simulink model "comprehensive_model_with_rocks_trial"  (R2019a)
settings: Solver=FixedStepAuto  StartTime=0.0  StopTime=15  FixedStep=0.001  RelTol=1e-3
PreLoadFcn:
  | load('tumbleweed_constants.mat')
values from neighbouring files (symbols this model uses):
  Ar = 0.785398163397    [tumbleweed_constants.mat]
  CD = 0.8    [tumbleweed_constants.mat]
  d = 0.65    [tumbleweed_constants.mat]
  g = 9.81    [tumbleweed_constants.mat]
  Ixx = 1.29    [tumbleweed_constants.mat]
  Iyy = 1.29    [tumbleweed_constants.mat]
  Izz = 1.29    [tumbleweed_constants.mat]
  m = 1    [tumbleweed_constants.mat]
  maxr = 0.45    [tumbleweed_constants.mat]
  mf = 14    [tumbleweed_constants.mat]
  minr = 0.2    [tumbleweed_constants.mat]
  mu0 = 0.02    [tumbleweed_constants.mat]
  muk = 0.5    [tumbleweed_constants.mat]
  must = 0.8    [tumbleweed_constants.mat]
  R = cylR*ones(size(Theta,1),size(Theta,2))    [d3_animate.m]    (also in tumbleweed_constants.mat = 0.5)
  rest_coeff = 0.6    [tumbleweed_constants.mat]
  rho = 1.2    [tumbleweed_constants.mat]
  ts = 0.5    [tumbleweed_constants.mat]
  v_thres = 0.0001    [tumbleweed_constants.mat]
  vmax = 0.2    [tumbleweed_constants.mat]
  YY = 50    [tumbleweed_constants.mat]
libraries: simulink x2
(part 1 of 9)
settings Model: Creator=racha  LastModifiedBy=racha

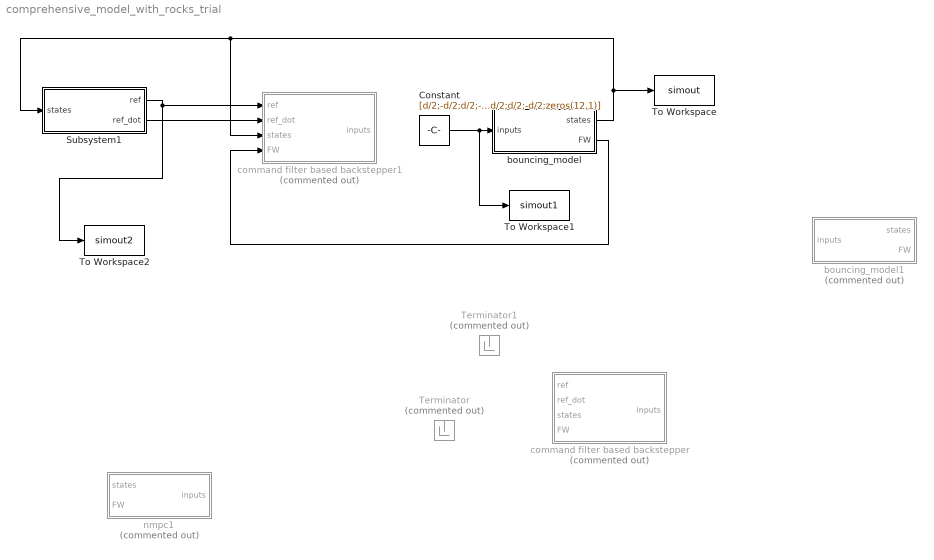
== system comprehensive_model_with_rocks_trial ==
  Constant : Constant  Value=[d/2;-d/2;d/2;-d/2;d/2;-d/2;zeros(12,1)]
  Subsystem1 : Subsystem
  Terminator : Terminator  Commented=on
  Terminator1 : Terminator  Commented=on
  To Workspace : ToWorkspace  VariableName=simout  SaveFormat=Timeseries  SampleTime=-1
  To Workspace1 : ToWorkspace  VariableName=simout1  SaveFormat=Timeseries  SampleTime=-1
  To Workspace2 : ToWorkspace  VariableName=simout2  SaveFormat=Timeseries  SampleTime=-1
  bouncing_model : Subsystem
  bouncing_model1 : Subsystem  Commented=on
  command filter based backstepper : Subsystem  Commented=on
  command filter based backstepper1 : Subsystem  Commented=on
  nmpc1 : Subsystem  Commented=on
  wires:
  bouncing_model/2(FW) -> command filter based backstepper1/4(FW)
  Subsystem1/1(ref) -> command filter based backstepper1/1(ref), To Workspace2/1
  Subsystem1/2("ref_dot ") -> command filter based backstepper1/2("ref_dot ")
  bouncing_model/1(states) -> command filter based backstepper1/3(states), Subsystem1/1(states), To Workspace/1
  Constant/1 -> To Workspace1/1, bouncing_model/1(inputs)

== system comprehensive_model_with_rocks_trial/Subsystem1 ==
  states : Inport
  Clock : Clock
  Constant : Constant  Commented=on  Value=[-0.5;-0.5;0.5]
  Data Store Memory : DataStoreMemory  DataStoreName=y_new  ReadBeforeWriteMsg=warning  WriteAfterWriteMsg=warning  WriteAfterReadMsg=warning  InitialValue=[0;0]  ShowAdditionalParam=off
  Data Store Memory1 : DataStoreMemory  DataStoreName=err  ReadBeforeWriteMsg=warning  WriteAfterWriteMsg=warning  WriteAfterReadMsg=warning  InitialValue=[0;0]  ShowAdditionalParam=off
  Data Store Memory2 : DataStoreMemory  DataStoreName=cum_err  ReadBeforeWriteMsg=warning  WriteAfterWriteMsg=warning  WriteAfterReadMsg=warning  ShowAdditionalParam=off
  Data Store Read : DataStoreRead  DataStoreName=hit
  Data Store Read1 : DataStoreRead  DataStoreName=y_new
  Data Store Read2 : DataStoreRead  DataStoreName=err
  Data Store Read3 : DataStoreRead  DataStoreName=cum_err
  Data Store Write : DataStoreWrite  DataStoreName=hit
  Data Store Write1 : DataStoreWrite  DataStoreName=y_new
  Data Store Write2 : DataStoreWrite  DataStoreName=err
  Data Store Write3 : DataStoreWrite  DataStoreName=cum_err
  MATLAB Function : MATLAB Function  TreatAsAtomicUnit=on
  Stop Simulation : Stop
  Uniform Random Number : UniformRandomNumber  Minimum=0  Seed=43  SampleTime=0.01
  t : DataStoreMemory  DataStoreName=hit  ReadBeforeWriteMsg=warning  WriteAfterWriteMsg=warning  WriteAfterReadMsg=warning  ShowAdditionalParam=off
  y_points : ToWorkspace  VariableName=simout5  SaveFormat=Timeseries  SampleTime=-1
  yref_points : ToWorkspace  VariableName=simout10  SaveFormat=Timeseries  SampleTime=-1
  ref : Outport
  "ref_dot " : Outport  Port=2
  wires:
  MATLAB Function/1(y) -> ref/1
  Clock/1 -> MATLAB Function/1(t)
  MATLAB Function/2(ydot) -> "ref_dot "/1
  states/1 -> MATLAB Function/2(states)
  Data Store Read/1 -> MATLAB Function/3("hit ")
  MATLAB Function/3(hit) -> Data Store Write/1
  Data Store Read1/1 -> MATLAB Function/4("y_new ")
  MATLAB Function/4(y_new) -> Data Store Write1/1, yref_points/1
  Data Store Read2/1 -> MATLAB Function/5("err ")
  Data Store Read3/1 -> MATLAB Function/6("cum_err ")
  MATLAB Function/5(err) -> y_points/1, Data Store Write2/1
  MATLAB Function/6(cum_err) -> Data Store Write3/1
  Uniform Random Number/1 -> MATLAB Function/7(rand_num)
  MATLAB Function/7(stop_flag) -> Stop Simulation/1

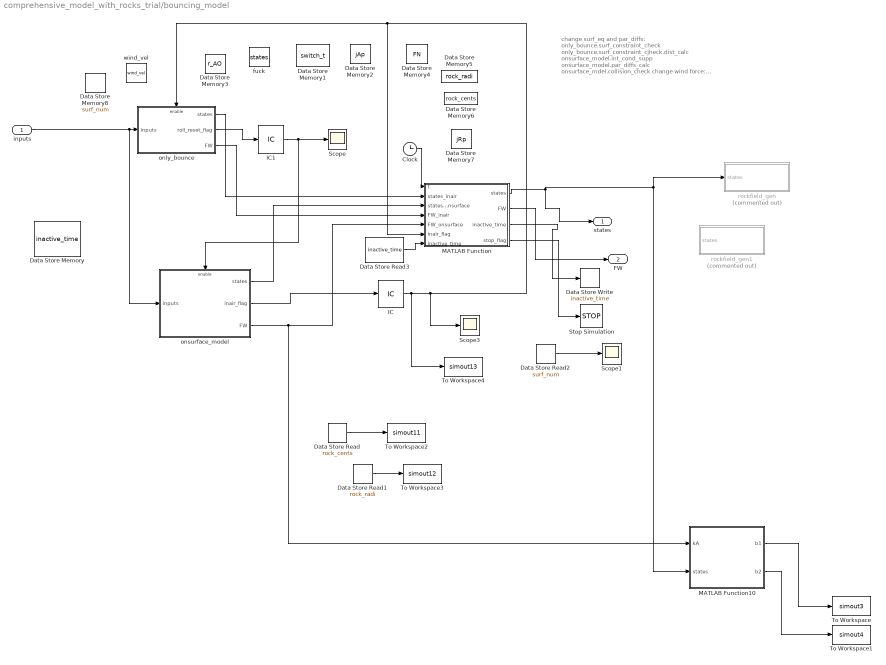
== system comprehensive_model_with_rocks_trial/bouncing_model ==
  note: change surf_eq and par_diffs:
      | only_bounce.surf_constraint_check
      | only_bounce.surf_constraint_cjheck.dist_calc
      | onsurface_model.int_cond_supp
      | onsurface_model.par_diffs_calc
      | onsurface_mdel.collision_check
      |
      | change wind force:
      | only_bounce.wind_force_calc
      | onsurface_model.wind_force_calc
      |
      | FN = 0 only when u start from surface
  inputs : Inport
  Clock : Clock
  Data Store Memory : DataStoreMemory  DataStoreName=inactive_time  ReadBeforeWriteMsg=warning  WriteAfterWriteMsg=warning  WriteAfterReadMsg=warning  ShowAdditionalParam=off
  Data Store Memory1 : DataStoreMemory  DataStoreName=switch_t  ReadBeforeWriteMsg=warning  WriteAfterWriteMsg=warning  WriteAfterReadMsg=warning  ShowAdditionalParam=off
  Data Store Memory2 : DataStoreMemory  DataStoreName=jAp  ReadBeforeWriteMsg=warning  WriteAfterWriteMsg=warning  WriteAfterReadMsg=warning  InitialValue=[0;1;0]  ShowAdditionalParam=off
  Data Store Memory3 : DataStoreMemory  DataStoreName=r_AO  ReadBeforeWriteMsg=warning  WriteAfterWriteMsg=warning  WriteAfterReadMsg=warning  InitialValue=[0;0;0]  ShowAdditionalParam=off
  Data Store Memory4 : DataStoreMemory  DataStoreName=FN  ReadBeforeWriteMsg=warning  WriteAfterWriteMsg=warning  WriteAfterReadMsg=warning  InitialValue=100  ShowAdditionalParam=off
  Data Store Memory5 : DataStoreMemory  DataStoreName=rock_radi  ReadBeforeWriteMsg=warning  WriteAfterWriteMsg=warning  WriteAfterReadMsg=warning  InitialValue=[0.2;0.5]  ShowAdditionalParam=off
  Data Store Memory6 : DataStoreMemory  DataStoreName=rock_cents  ReadBeforeWriteMsg=warning  WriteAfterWriteMsg=warning  WriteAfterReadMsg=warning  InitialValue=[5,7;0,0;-0.1,-0.1]  ShowAdditionalParam=off
  Data Store Memory7 : DataStoreMemory  DataStoreName=jRp  ReadBeforeWriteMsg=warning  WriteAfterWriteMsg=warning  WriteAfterReadMsg=warning  InitialValue=[0;1;0]  ShowAdditionalParam=off
  Data Store Memory8 : DataStoreMemory  DataStoreName=surf_num  ReadBeforeWriteMsg=warning  WriteAfterWriteMsg=warning  WriteAfterReadMsg=warning  ShowAdditionalParam=off
  Data Store Read : DataStoreRead  DataStoreName=rock_cents
  Data Store Read1 : DataStoreRead  DataStoreName=rock_radi
  Data Store Read2 : DataStoreRead  DataStoreName=surf_num
  Data Store Read3 : DataStoreRead  DataStoreName=inactive_time
  Data Store Write : DataStoreWrite  DataStoreName=inactive_time
  IC : InitialCondition
  IC1 : InitialCondition  Value=0
  MATLAB Function : MATLAB Function  TreatAsAtomicUnit=on
  MATLAB Function10 : MATLAB Function  TreatAsAtomicUnit=on
  Scope : Scope
  Scope1 : Scope
  Scope3 : Scope
  Stop Simulation : Stop
  To Workspace : ToWorkspace  VariableName=simout3  SaveFormat=Timeseries  SampleTime=-1
  To Workspace1 : ToWorkspace  VariableName=simout4  SaveFormat=Timeseries  SampleTime=-1
  To Workspace2 : ToWorkspace  VariableName=simout11  SaveFormat=Timeseries  SampleTime=-1
  To Workspace3 : ToWorkspace  VariableName=simout12  SaveFormat=Timeseries  SampleTime=-1
  To Workspace4 : ToWorkspace  VariableName=simout13  SaveFormat=Timeseries  SampleTime=-1
  fuck : DataStoreMemory  DataStoreName=states  ReadBeforeWriteMsg=warning  WriteAfterWriteMsg=warning  WriteAfterReadMsg=warning  InitialValue=[0;0.0001;0;7;0;0;0;0;R;1;0;0;0]  ShowAdditionalParam=off
  only_bounce : Subsystem
  onsurface_model : Subsystem
  rockfield_gen : Subsystem  Commented=on
  rockfield_gen1 : Subsystem  Commented=on
  wind_vel : DataStoreMemory  DataStoreName=wind_vel  ReadBeforeWriteMsg=warning  WriteAfterWriteMsg=warning  WriteAfterReadMsg=warning  ShowAdditionalParam=off
  states : Outport
  FW : Outport  Port=2
  wires:
  only_bounce/2(roll_reset_flag) -> IC1/1
  onsurface_model/2(inair_flag) -> IC/1
  IC/1 -> To Workspace4/1, Scope3/1, MATLAB Function/6(inair_flag), only_bounce/Enable
  inputs/1 -> onsurface_model/1("inputs "), only_bounce/1(inputs)
  IC1/1 -> onsurface_model/Enable, Scope/1
  only_bounce/1(states) -> MATLAB Function/2(states_inair)
  onsurface_model/1(states) -> MATLAB Function/3(states_onsurface)
  only_bounce/3(FW) -> MATLAB Function/4(FW_inair)
  MATLAB Function/2(FW) -> FW/1
  Data Store Read2/1 -> Scope1/1
  MATLAB Function10/2(b2) -> To Workspace1/1
  MATLAB Function/1(states) -> states/1, rockfield_gen/1(states), MATLAB Function10/2(states)
  MATLAB Function10/1(b1) -> To Workspace/1
  Data Store Read/1 -> To Workspace2/1
  Data Store Read1/1 -> To Workspace3/1
  Data Store Read3/1 -> MATLAB Function/7("inactive_time ")
  MATLAB Function/3(inactive_time) -> Data Store Write/1
  MATLAB Function/4(stop_flag) -> Stop Simulation/1
  Clock/1 -> MATLAB Function/1(t)
  onsurface_model/3(FW) -> MATLAB Function/5(FW_onsurface), MATLAB Function10/1(kA)

== system comprehensive_model_with_rocks_trial/bouncing_model1 ==
  note: change surf_eq and par_diffs:
      | only_bounce.surf_constraint_check
      | only_bounce.surf_constraint_cjheck.dist_calc
      | onsurface_model.int_cond_supp
      | onsurface_model.par_diffs_calc
      | onsurface_mdel.collision_check
      |
      | change wind force:
      | only_bounce.wind_force_calc
      | onsurface_model.wind_force_calc
      |
      | FN = 0 only when u start from surface
  inputs : Inport
  Data Store Memory : DataStoreMemory  DataStoreName=states  ReadBeforeWriteMsg=warning  WriteAfterWriteMsg=warning  WriteAfterReadMsg=warning  InitialValue=[0;0.5653/R;0;0.5653;0;0;0;0;R;1;0;0;0]  ShowAdditionalParam=off
  Data Store Memory1 : DataStoreMemory  DataStoreName=switch_t  ReadBeforeWriteMsg=warning  WriteAfterWriteMsg=warning  WriteAfterReadMsg=warning  ShowAdditionalParam=off
  Data Store Memory2 : DataStoreMemory  DataStoreName=jAp  ReadBeforeWriteMsg=warning  WriteAfterWriteMsg=warning  WriteAfterReadMsg=warning  InitialValue=[0;1;0]  ShowAdditionalParam=off
  Data Store Memory3 : DataStoreMemory  DataStoreName=r_AO  ReadBeforeWriteMsg=warning  WriteAfterWriteMsg=warning  WriteAfterReadMsg=warning  InitialValue=[0;0;0]  ShowAdditionalParam=off
  Data Store Memory4 : DataStoreMemory  DataStoreName=FN  ReadBeforeWriteMsg=warning  WriteAfterWriteMsg=warning  WriteAfterReadMsg=warning  ShowAdditionalParam=off
  Data Store Memory5 : DataStoreMemory  DataStoreName=rock_radi  ReadBeforeWriteMsg=warning  WriteAfterWriteMsg=warning  WriteAfterReadMsg=warning  InitialValue=[0.2;0.5]  ShowAdditionalParam=off
  Data Store Memory6 : DataStoreMemory  DataStoreName=rock_cents  ReadBeforeWriteMsg=warning  WriteAfterWriteMsg=warning  WriteAfterReadMsg=warning  InitialValue=[5,7; 10,10; -0.1,-0.1]  ShowAdditionalParam=off
  Data Store Memory7 : DataStoreMemory  DataStoreName=jRp  ReadBeforeWriteMsg=warning  WriteAfterWriteMsg=warning  WriteAfterReadMsg=warning  InitialValue=[0;1;0]  ShowAdditionalParam=off
  Data Store Memory8 : DataStoreMemory  DataStoreName=surf_num  ReadBeforeWriteMsg=warning  WriteAfterWriteMsg=warning  WriteAfterReadMsg=warning  ShowAdditionalParam=off
  Data Store Memory9 : DataStoreMemory  DataStoreName=wind_vel  ReadBeforeWriteMsg=warning  WriteAfterWriteMsg=warning  WriteAfterReadMsg=warning  ShowAdditionalParam=off
  Data Store Read : DataStoreRead  DataStoreName=rock_cents
  Data Store Read1 : DataStoreRead  DataStoreName=rock_radi
  Data Store Read2 : DataStoreRead  DataStoreName=surf_num
  IC : InitialCondition
  IC1 : InitialCondition  Value=0
  MATLAB Function : MATLAB Function  TreatAsAtomicUnit=on
  Scope : Scope
  Scope1 : Scope
  Scope3 : Scope
  To Workspace : ToWorkspace  VariableName=simout7  SaveFormat=Timeseries  SampleTime=-1
  To Workspace1 : ToWorkspace  VariableName=simout8  SaveFormat=Timeseries  SampleTime=-1
  only_bounce : Subsystem
  onsurface_model : Subsystem
  states : Outport
  FW : Outport  Port=2
  wires:
  only_bounce/2(roll_reset_flag) -> IC1/1
  onsurface_model/2(inair_flag) -> IC/1
  IC/1 -> Scope3/1, MATLAB Function/5(inair_flag), only_bounce/Enable
  inputs/1 -> onsurface_model/1("inputs "), only_bounce/1(inputs)
  IC1/1 -> onsurface_model/Enable, Scope/1
  only_bounce/1(states) -> MATLAB Function/1(states_inair)
  onsurface_model/1(states) -> MATLAB Function/2(states_onsurface)
  MATLAB Function/1(states) -> states/1
  only_bounce/3(FW) -> MATLAB Function/3(FW_inair)
  onsurface_model/3(FW) -> MATLAB Function/4(FW_onsurface)
  MATLAB Function/2(FW) -> FW/1
  Data Store Read/1 -> To Workspace/1
  Data Store Read1/1 -> To Workspace1/1
  Data Store Read2/1 -> Scope1/1

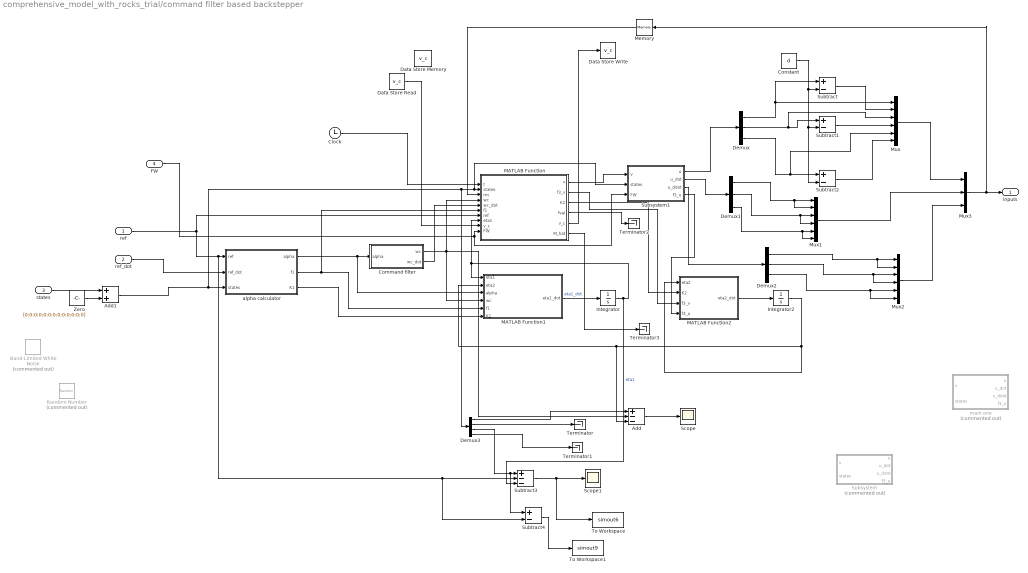
== system comprehensive_model_with_rocks_trial/command filter based backstepper ==
  ref : Inport
  "ref_dot " : Inport  Port=2
  states : Inport  Port=3
  FW : Inport  Port=4
  Add : Sum  Inputs=+--
  Add1 : Sum
  Band-Limited White Noise : simulink/Sources/Band-Limited White Noise  Commented=on  Cov=[0.002;0.002;0.002;0.002;0.002;0.001;0.05;0.05;0.05;0.001;0.001;0.001;0.001]  Ts=0.001  seed=[23340]
  Clock : Clock
  Command filter : Subsystem
  Constant : Constant  Value=d
  Data Store Memory : DataStoreMemory  DataStoreName=v_c  ReadBeforeWriteMsg=warning  WriteAfterWriteMsg=warning  WriteAfterReadMsg=warning  InitialValue=[0.325;0.325;0.325;0]  ShowAdditionalParam=off
  Data Store Read : DataStoreRead  DataStoreName=v_c
  Data Store Write : DataStoreWrite  DataStoreName=v_c
  Demux : Demux  Outputs=3
  Demux1 : Demux  Outputs=3
  Demux2 : Demux  Outputs=3
  Demux3 : Demux  Outputs=[3;3;3;4]
  Integrator : Integrator  InitialCondition=[0;0;0]
  Integrator2 : Integrator  InitialCondition=[0;0;0]
  MATLAB Function : MATLAB Function  TreatAsAtomicUnit=on
  MATLAB Function1 : MATLAB Function  TreatAsAtomicUnit=on
  MATLAB Function2 : MATLAB Function  TreatAsAtomicUnit=on
  Memory : Memory  InitialCondition=[d/2;-d/2;d/2;-d/2;d/2;-d/2;0;0;0;0;0;0;0;0;0;0;0;0]
  Mux : Mux  Inputs=6
  Mux1 : Mux  Inputs=6
  Mux2 : Mux  Inputs=6
  Mux3 : Mux  Inputs=3
  Random Number : RandomNumber  Commented=on  Mean=zeros(13,1)  Variance=[0.1;0.1;0.1;0.1;0.1;0.1;0.2;0.2;0.2;0.01;0.01;0.01;0.01]  Seed=randi(1000,13,1)  SampleTime=0.001
  Scope : Scope
  Scope1 : Scope
  Subsystem : Subsystem  Commented=on
  Subsystem1 : Subsystem
  Subtract{,1..2,4} (4 alike) : Sum  Inputs=+-
  Subtract3 : Sum  Inputs=+--
  Terminator{,1..3} (4 alike) : Terminator
  To Workspace : ToWorkspace  VariableName=simout6  SaveFormat=Timeseries  SampleTime=-1
  To Workspace1 : ToWorkspace  VariableName=simout9  SaveFormat=Timeseries  SampleTime=-1
  Zero : Constant  Value=[0;0;0;0;0;0;0;0;0;0;0;0;0]  OutDataTypeStr=Inherit: Inherit via back propagation
  alpha calculator : MATLAB Function  TreatAsAtomicUnit=on
  main one : Subsystem  Commented=on
  inputs : Outport
  wires:
  alpha calculator/1(alpha) -> Command filter/1(alpha), MATLAB Function1/3(alpha)
  MATLAB Function1/1(eta1_dot) -> Integrator/1  "eta1_dot"
  Integrator/1 -> Subtract3/3, MATLAB Function/8(eta1), MATLAB Function1/1(eta1)  "eta1"
  alpha calculator/2(f1) -> MATLAB Function/6(f1), MATLAB Function1/5(f1)
  alpha calculator/3(K1) -> MATLAB Function1/6(K1)
  ref/1 -> MATLAB Function/7(ref), Subtract4/2, Subtract3/2, alpha calculator/1(ref)
  "ref_dot "/1 -> alpha calculator/2(ref_dot)
  Command filter/2(wc_dot) -> MATLAB Function/5(wc_dot)
  Command filter/1(wc) -> MATLAB Function/4(wc), MATLAB Function1/4(wc), Add/2
  MATLAB Function/1(v) -> Subsystem1/1(v)
  Subsystem1/1(u) -> Demux/1
  Subsystem1/2(u_dot) -> Demux1/1
  Mux3/1 -> Memory/1, inputs/1
  MATLAB Function/3(K2) -> MATLAB Function2/2(K2)
  MATLAB Function/2(f3_v) -> MATLAB Function2/3(f3_v)
  Subsystem1/4(f3_u) -> MATLAB Function2/4(f3_u)
  MATLAB Function2/1(eta2_dot) -> Integrator2/1
  Integrator2/1 -> MATLAB Function1/2(eta2), Add/3, MATLAB Function2/1(eta2)
  Subsystem1/3(u_ddot) -> Demux2/1
  Demux/3 -> Mux/5, Subtract2/1
  Demux/2 -> Mux/3, Subtract1/1
  Demux/1 -> Mux/1, Subtract/1
  Constant/1 -> Subtract2/2, Subtract1/2, Subtract/2
  Subtract/1 -> Mux/2
  Subtract1/1 -> Mux/4
  Subtract2/1 -> Mux/6
  Mux/1 -> Mux3/1
  Demux1/1 -> Mux1/2, Mux1/1
  Demux1/2 -> Mux1/4, Mux1/3
  Demux1/3 -> Mux1/6, Mux1/5
  Demux2/3 -> Mux2/6, Mux2/5
  Demux2/1 -> Mux2/2, Mux2/1
  Demux2/2 -> Mux2/4, Mux2/3
  Mux1/1 -> Mux3/2
  Mux2/1 -> Mux3/3
  Memory/1 -> MATLAB Function/3(rm)
  Clock/1 -> MATLAB Function/1(t)
  MATLAB Function/4(fval) -> Terminator2/1
  Data Store Read/1 -> MATLAB Function/9("v_c ")
  MATLAB Function/5(v_c) -> Data Store Write/1
  MATLAB Function/6(M_hat) -> Terminator3/1
  Demux3/2 -> Terminator/1
  Demux3/1 -> Add/1
  Add/1 -> Scope/1
  Demux3/4 -> Terminator1/1
  Demux3/3 -> Subtract4/1, Subtract3/1
  Subtract3/1 -> To Workspace/1, Scope1/1
  Add1/1 -> Demux3/1, Subsystem1/2(states), MATLAB Function/2(states), alpha calculator/3(states)
  states/1 -> Add1/1
  Zero/1 -> Add1/2
  FW/1 -> Subsystem1/3(FW), MATLAB Function/10(FW)
  Subtract4/1 -> To Workspace1/1

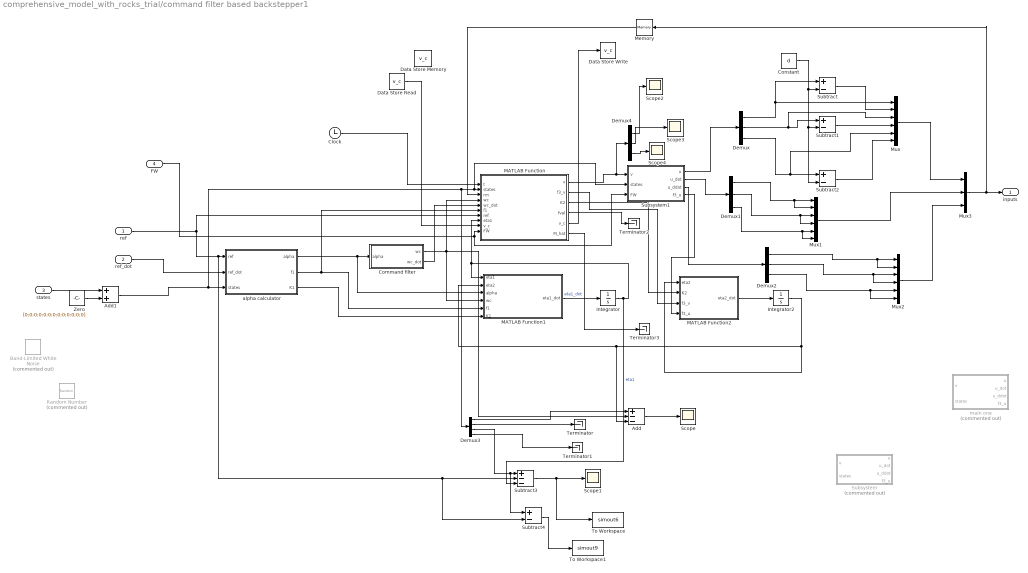
== system comprehensive_model_with_rocks_trial/command filter based backstepper1 ==
  ref : Inport
  "ref_dot " : Inport  Port=2
  states : Inport  Port=3
  FW : Inport  Port=4
  Add : Sum  Inputs=+--
  Add1 : Sum
  Band-Limited White Noise : simulink/Sources/Band-Limited White Noise  Commented=on  Cov=[0.002;0.002;0.002;0.002;0.002;0.001;0.05;0.05;0.05;0.001;0.001;0.001;0.001]  Ts=0.001  seed=[23340]
  Clock : Clock
  Command filter : Subsystem
  Constant : Constant  Value=d
  Data Store Memory : DataStoreMemory  DataStoreName=v_c  ReadBeforeWriteMsg=warning  WriteAfterWriteMsg=warning  WriteAfterReadMsg=warning  InitialValue=[0.325;0.325;0.325;0]  ShowAdditionalParam=off
  Data Store Read : DataStoreRead  DataStoreName=v_c
  Data Store Write : DataStoreWrite  DataStoreName=v_c
  Demux{,1..2,4} (4 alike) : Demux  Outputs=3
  Demux3 : Demux  Outputs=[3;3;3;4]
  Integrator : Integrator  InitialCondition=[0;0;0]
  Integrator2 : Integrator  InitialCondition=[0;0;0]
  MATLAB Function : MATLAB Function  TreatAsAtomicUnit=on
  MATLAB Function1 : MATLAB Function  TreatAsAtomicUnit=on
  MATLAB Function2 : MATLAB Function  TreatAsAtomicUnit=on
  Memory : Memory  InitialCondition=[d/2;-d/2;d/2;-d/2;d/2;-d/2;0;0;0;0;0;0;0;0;0;0;0;0]
  Mux : Mux  Inputs=6
  Mux1 : Mux  Inputs=6
  Mux2 : Mux  Inputs=6
  Mux3 : Mux  Inputs=3
  Random Number : RandomNumber  Commented=on  Mean=zeros(13,1)  Variance=[0.1;0.1;0.1;0.1;0.1;0.1;0.2;0.2;0.2;0.01;0.01;0.01;0.01]  Seed=randi(1000,13,1)  SampleTime=0.001
  Scope{,1..4} (5 alike) : Scope
  Subsystem : Subsystem  Commented=on
  Subsystem1 : Subsystem
  Subtract{,1..2,4} (4 alike) : Sum  Inputs=+-
  Subtract3 : Sum  Inputs=+--
  Terminator{,1..3} (4 alike) : Terminator
  To Workspace : ToWorkspace  VariableName=simout6  SaveFormat=Timeseries  SampleTime=-1
  To Workspace1 : ToWorkspace  VariableName=simout9  SaveFormat=Timeseries  SampleTime=-1
  Zero : Constant  Value=[0;0;0;0;0;0;0;0;0;0;0;0;0]  OutDataTypeStr=Inherit: Inherit via back propagation
  alpha calculator : MATLAB Function  TreatAsAtomicUnit=on
  main one : Subsystem  Commented=on
  inputs : Outport
  wires:
  alpha calculator/1(alpha) -> Command filter/1(alpha), MATLAB Function1/3(alpha)
  MATLAB Function1/1(eta1_dot) -> Integrator/1  "eta1_dot"
  Integrator/1 -> Subtract3/3, MATLAB Function/8(eta1), MATLAB Function1/1(eta1)  "eta1"
  alpha calculator/2(f1) -> MATLAB Function/6(f1), MATLAB Function1/5(f1)
  alpha calculator/3(K1) -> MATLAB Function1/6(K1)
  ref/1 -> MATLAB Function/7(ref), Subtract4/2, Subtract3/2, alpha calculator/1(ref)
  "ref_dot "/1 -> alpha calculator/2(ref_dot)
  Command filter/2(wc_dot) -> MATLAB Function/5(wc_dot)
  Command filter/1(wc) -> MATLAB Function/4(wc), MATLAB Function1/4(wc), Add/2
  MATLAB Function/1(v) -> Demux4/1, Subsystem1/1(v)
  Subsystem1/1(u) -> Demux/1
  Subsystem1/2(u_dot) -> Demux1/1
  Mux3/1 -> Memory/1, inputs/1
  MATLAB Function/3(K2) -> MATLAB Function2/2(K2)
  MATLAB Function/2(f3_v) -> MATLAB Function2/3(f3_v)
  Subsystem1/4(f3_u) -> MATLAB Function2/4(f3_u)
  MATLAB Function2/1(eta2_dot) -> Integrator2/1
  Integrator2/1 -> MATLAB Function1/2(eta2), Add/3, MATLAB Function2/1(eta2)
  Subsystem1/3(u_ddot) -> Demux2/1
  Demux/3 -> Mux/5, Subtract2/1
  Demux/2 -> Mux/3, Subtract1/1
  Demux/1 -> Mux/1, Subtract/1
  Constant/1 -> Subtract2/2, Subtract1/2, Subtract/2
  Subtract/1 -> Mux/2
  Subtract1/1 -> Mux/4
  Subtract2/1 -> Mux/6
  Mux/1 -> Mux3/1
  Demux1/1 -> Mux1/2, Mux1/1
  Demux1/2 -> Mux1/4, Mux1/3
  Demux1/3 -> Mux1/6, Mux1/5
  Demux2/3 -> Mux2/6, Mux2/5
  Demux2/1 -> Mux2/2, Mux2/1
  Demux2/2 -> Mux2/4, Mux2/3
  Mux1/1 -> Mux3/2
  Mux2/1 -> Mux3/3
  Memory/1 -> MATLAB Function/3(rm)
  Clock/1 -> MATLAB Function/1(t)
  MATLAB Function/4(fval) -> Terminator2/1
  Data Store Read/1 -> MATLAB Function/9("v_c ")
  MATLAB Function/5(v_c) -> Data Store Write/1
  MATLAB Function/6(M_hat) -> Terminator3/1
  Demux3/2 -> Terminator/1
  Demux3/1 -> Add/1
  Add/1 -> Scope/1
  Demux3/4 -> Terminator1/1
  Demux3/3 -> Subtract4/1, Subtract3/1
  Subtract3/1 -> To Workspace/1, Scope1/1
  Add1/1 -> Demux3/1, Subsystem1/2(states), MATLAB Function/2(states), alpha calculator/3(states)
  states/1 -> Add1/1
  Zero/1 -> Add1/2
  FW/1 -> Subsystem1/3(FW), MATLAB Function/10(FW)
  Subtract4/1 -> To Workspace1/1
  Demux4/1 -> Scope2/1
  Demux4/2 -> Scope3/1
  Demux4/3 -> Scope4/1

== system comprehensive_model_with_rocks_trial/nmpc1 ==
  states : Inport
  FW : Inport  Port=2
  Clock : Clock
  Constant : Constant  Value=[0;0;0]
  Constant1 : Constant  Value=d
  Data Store Memory : DataStoreMemory  DataStoreName=u_dot_c  ReadBeforeWriteMsg=warning  WriteAfterWriteMsg=warning  WriteAfterReadMsg=warning  InitialValue=zeros(3,4)  ShowAdditionalParam=off
  Data Store Memory1 : DataStoreMemory  DataStoreName=idx  ReadBeforeWriteMsg=warning  WriteAfterWriteMsg=warning  WriteAfterReadMsg=warning  InitialValue=1  ShowAdditionalParam=off
  Data Store Read : DataStoreRead  DataStoreName=idx
  Data Store Read2 : DataStoreRead  DataStoreName=u_dot_c
  Data Store Write : DataStoreWrite  DataStoreName=u_dot_c
  Data Store Write2 : DataStoreWrite  DataStoreName=idx
  Demux : Demux  Outputs=3
  Demux1 : Demux  Outputs=3
  Demux2 : Demux  Outputs=3
  Integrator : Integrator  InitialCondition=[0.325;0.325;0.325]
  MATLAB Function1 : MATLAB Function  TreatAsAtomicUnit=on
  Memory : Memory  InitialCondition=[d/2;-d/2;d/2;-d/2;d/2;-d/2;zeros(12,1)]
  Mux : Mux  Inputs=6
  Mux1 : Mux  Inputs=6
  Mux2 : Mux  Inputs=3
  Mux3 : Mux  Inputs=6
  Subtract : Sum  Inputs=+-
  Subtract1 : Sum  Inputs=+-
  Subtract2 : Sum  Inputs=+-
  u_dot generator : MATLAB Function  TreatAsAtomicUnit=on
  inputs : Outport
  wires:
  states/1 -> u_dot generator/2(states)
  Clock/1 -> MATLAB Function1/1(t), u_dot generator/1(t)
  Memory/1 -> MATLAB Function1/2(rm), u_dot generator/3(rm), inputs/1
  Integrator/1 -> Demux/1
  MATLAB Function1/2(idx_n) -> Data Store Write2/1
  u_dot generator/1(udotc) -> MATLAB Function1/3(udot_mat), Data Store Write/1
  u_dot generator/2(idxn) -> MATLAB Function1/4(idx)
  Data Store Read2/1 -> u_dot generator/5(udot_mat)
  Data Store Read/1 -> u_dot generator/6(idx)
  Demux/1 -> Mux/1, Subtract/1
  Constant1/1 -> Subtract2/2, Subtract1/2, Subtract/2
  Subtract1/1 -> Mux/4
  Demux/2 -> Mux/3, Subtract1/1
  Mux/1 -> Mux2/1
  Subtract2/1 -> Mux/6
  Demux/3 -> Mux/5, Subtract2/1
  Subtract/1 -> Mux/2
  Demux1/1 -> Mux1/2, Mux1/1
  Mux1/1 -> Mux2/2
  MATLAB Function1/1(udot) -> Demux1/1, Integrator/1
  Demux1/3 -> Mux1/6, Mux1/5
  Demux1/2 -> Mux1/4, Mux1/3
  Constant/1 -> Demux2/1
  Demux2/2 -> Mux3/3, Mux3/4
  Demux2/3 -> Mux3/6, Mux3/5
  Mux3/1 -> Mux2/3
  Demux2/1 -> Mux3/1, Mux3/2
  Mux2/1 -> Memory/1
  FW/1 -> u_dot generator/4(FW)

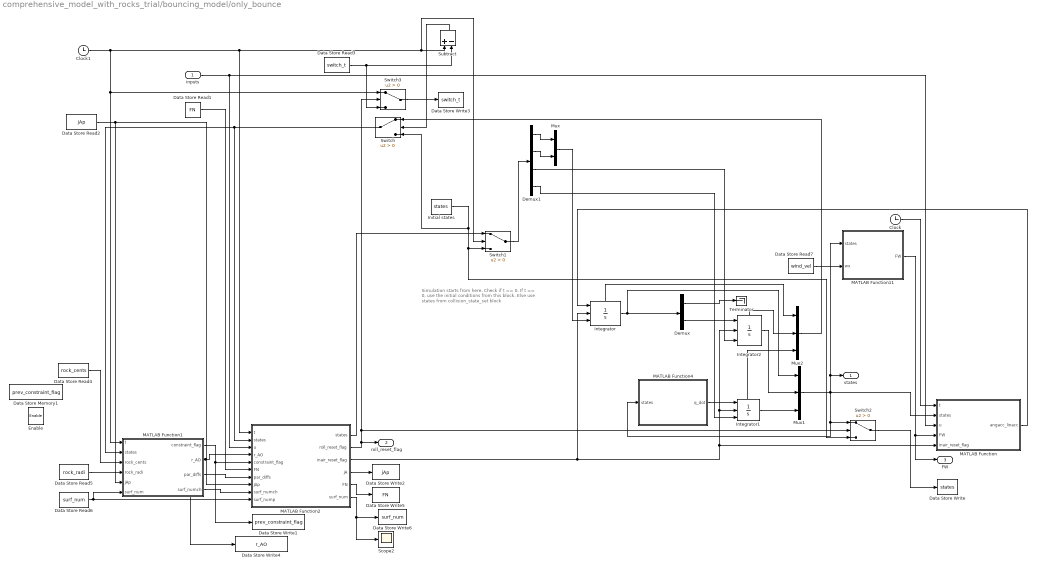
== system comprehensive_model_with_rocks_trial/bouncing_model/only_bounce ==
  note: Simulation starts from here.
      | Check if t == 0.
      | If t == 0, use the initial conditions from this block.
      | Else use states from collision_state_set block
  inputs : Inport
  Enable : EnablePort  StatesWhenEnabling=reset
  Clock : Clock
  Clock1 : Clock
  Data Store Memory1 : DataStoreMemory  DataStoreName=prev_constraint_flag  ReadBeforeWriteMsg=warning  WriteAfterWriteMsg=warning  WriteAfterReadMsg=warning  ShowAdditionalParam=off
  Data Store Read1 : DataStoreRead  DataStoreName=FN
  Data Store Read2 : DataStoreRead  DataStoreName=jAp
  Data Store Read3 : DataStoreRead  DataStoreName=switch_t
  Data Store Read4 : DataStoreRead  DataStoreName=rock_cents
  Data Store Read5 : DataStoreRead  DataStoreName=rock_radi
  Data Store Read6 : DataStoreRead  DataStoreName=surf_num
  Data Store Read7 : DataStoreRead  DataStoreName=wind_vel
  Data Store Write : DataStoreWrite  DataStoreName=states
  Data Store Write1 : DataStoreWrite  DataStoreName=prev_constraint_flag
  Data Store Write2 : DataStoreWrite  DataStoreName=jAp
  Data Store Write3 : DataStoreWrite  DataStoreName=switch_t
  Data Store Write4 : DataStoreWrite  DataStoreName=r_AO
  Data Store Write5 : DataStoreWrite  DataStoreName=FN
  Data Store Write6 : DataStoreWrite  DataStoreName=surf_num
  Demux : Demux  Outputs=[3;3]
  Demux1 : Demux  Outputs=[3;3;3;4]
  Initial states : DataStoreRead  DataStoreName=states
  Integrator : Integrator  ExternalReset=level hold  InitialConditionSource=external  ShowStatePort=on
  Integrator1 : Integrator  ExternalReset=level hold  InitialConditionSource=external  ShowStatePort=on
  Integrator2 : Integrator  ExternalReset=level hold  InitialConditionSource=external  ShowStatePort=on
  MATLAB Function : MATLAB Function  TreatAsAtomicUnit=on
  MATLAB Function1 : MATLAB Function  TreatAsAtomicUnit=on
  MATLAB Function11 : MATLAB Function  TreatAsAtomicUnit=on
  MATLAB Function2 : MATLAB Function  TreatAsAtomicUnit=on
  MATLAB Function4 : MATLAB Function  TreatAsAtomicUnit=on
  Mux : Mux  Inputs=2
  Mux1 : Mux  Inputs=[6;3;4]
  Mux2 : Mux  Inputs=[6;3;4]
  Scope2 : Scope
  Subtract : Sum  Inputs=+-
  Switch{,1..3} (4 alike) : Switch  Criteria=u2 > Threshold
  Terminator : Terminator
  states : Outport  SourceOfInitialOutputValue=Input signal  InitialOutput=zeros(13,1)
  roll_reset_flag : Outport  Port=2  InitialOutput=0
  FW : Outport  Port=3
  wires:
  MATLAB Function2/5(FN) -> Data Store Write5/1
  Demux1/3 -> Integrator2/3
  Data Store Read7/1 -> MATLAB Function11/2(wx)
  Switch3/1 -> Data Store Write3/1
  MATLAB Function1/4(surf_numch) -> MATLAB Function2/9(surf_numch)
  MATLAB Function1/3(par_diffs) -> MATLAB Function2/7(par_diffs)
  Data Store Read5/1 -> MATLAB Function1/4(rock_radi)
  Data Store Read4/1 -> MATLAB Function1/3(rock_cents)
  Subtract/1 -> Switch/2
  Data Store Read1/1 -> MATLAB Function2/6("FN ")
  Switch2/1 -> Data Store Write/1
  MATLAB Function2/1(states) -> Switch1/1
  Mux2/1 -> Switch/1
  Integrator2/1 -> Mux1/2
  MATLAB Function/1(angacc_linacc) -> Integrator/1
  Demux1/1 -> Mux/1
  Mux/1 -> Integrator/3
  Integrator1/State -> Mux2/3
  Demux/2 -> Integrator2/1
  MATLAB Function1/1(constraint_flag) -> MATLAB Function2/5(constraint_flag), Data Store Write1/1
  Switch1/1 -> Demux1/1
  Demux/1 -> Terminator/1
  Demux1/4 -> Integrator1/3
  Demux1/2 -> Mux/2
  Data Store Read2/1 -> MATLAB Function1/5(jAp), MATLAB Function2/8(jAp)
  Clock/1 -> MATLAB Function/1(t)
  Integrator1/1 -> Mux1/3
  MATLAB Function4/1(q_dot) -> Integrator1/1
  Integrator/State -> Mux2/1
  MATLAB Function2/4(jA) -> Data Store Write2/1
  Integrator2/State -> Mux2/2
  Data Store Read6/1 -> MATLAB Function1/6(surf_num), MATLAB Function2/10(surf_nump)
  MATLAB Function2/6(surf_num) -> Scope2/1, Data Store Write6/1
  MATLAB Function2/2(roll_reset_flag) -> Switch2/2, Switch3/2, roll_reset_flag/1
  Data Store Read3/1 -> Switch3/3, Subtract/2
  Initial states/1 -> Switch2/3, Switch1/3, Switch/3
  Switch/1 -> MATLAB Function2/2("states "), MATLAB Function1/2(states)
  MATLAB Function11/1(FW) -> MATLAB Function/4(FW), FW/1
  MATLAB Function1/2(r_AO) -> Data Store Write4/1, MATLAB Function2/4(r_AO)
  MATLAB Function2/3(inair_reset_flag) -> Integrator2/2, Integrator1/2, MATLAB Function/5(inair_reset_flag), Integrator/2
  inputs/1 -> MATLAB Function/3(u), MATLAB Function2/3(u)
  Integrator/1 -> Mux1/1, Demux/1
  Mux1/1 -> MATLAB Function4/1(states), Switch2/1, MATLAB Function11/1(states), states/1, MATLAB Function/2(states)
  Clock1/1 -> MATLAB Function1/1(t), Switch3/1, Subtract/1, Switch1/2, MATLAB Function2/1(t)

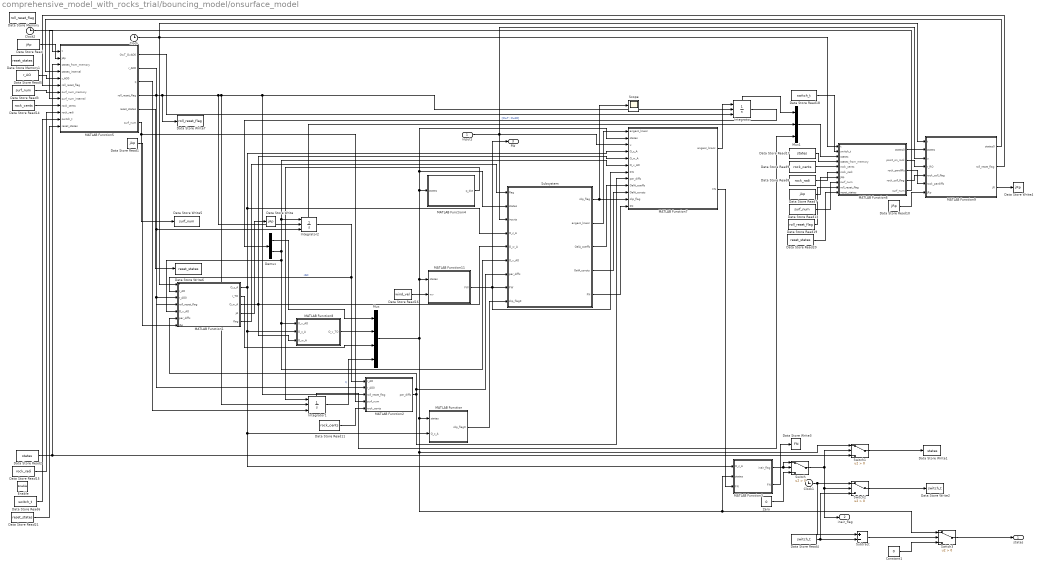
== system comprehensive_model_with_rocks_trial/bouncing_model/onsurface_model ==
  "inputs " : Inport
  Enable : EnablePort  StatesWhenEnabling=reset
  Clock : Clock
  Clock1 : Clock
  Clock2 : Clock
  Constant1 : Constant  Value=0  VectorParams1D=off
  Data Store Memory : DataStoreMemory  DataStoreName=roll_reset_flag  ReadBeforeWriteMsg=warning  WriteAfterWriteMsg=warning  WriteAfterReadMsg=warning  ShowAdditionalParam=off
  Data Store Memory1 : DataStoreMemory  DataStoreName=reset_states  ReadBeforeWriteMsg=warning  WriteAfterWriteMsg=warning  WriteAfterReadMsg=warning  InitialValue=zeros(13,1)  ShowAdditionalParam=off
  Data Store Read : DataStoreRead  DataStoreName=jAp
  Data Store Read1 : DataStoreRead  DataStoreName=jAp
  Data Store Read10 : DataStoreRead  DataStoreName=jRp
  Data Store Read11 : DataStoreRead  DataStoreName=rock_cents
  Data Store Read13 : DataStoreRead  DataStoreName=surf_num
  Data Store Read14 : DataStoreRead  DataStoreName=rock_cents
  Data Store Read15 : DataStoreRead  DataStoreName=rock_radi
  Data Store Read16 : DataStoreRead  DataStoreName=wind_vel
  Data Store Read17 : DataStoreRead  DataStoreName=states
  Data Store Read18 : DataStoreRead  DataStoreName=switch_t
  Data Store Read19 : DataStoreRead  DataStoreName=roll_reset_flag
  Data Store Read2 : DataStoreRead  DataStoreName=states
  Data Store Read20 : DataStoreRead  DataStoreName=reset_states
  Data Store Read21 : DataStoreRead  DataStoreName=reset_states
  Data Store Read3 : DataStoreRead  DataStoreName=surf_num
  Data Store Read4 : DataStoreRead  DataStoreName=switch_t
  Data Store Read5 : DataStoreRead  DataStoreName=r_AO
  Data Store Read6 : DataStoreRead  DataStoreName=switch_t
  Data Store Read7 : DataStoreRead  DataStoreName=jAp
  Data Store Read8 : DataStoreRead  DataStoreName=rock_radi
  Data Store Read9 : DataStoreRead  DataStoreName=rock_cents
  Data Store Write : DataStoreWrite  DataStoreName=jAp
  Data Store Write1 : DataStoreWrite  DataStoreName=states
  Data Store Write2 : DataStoreWrite  DataStoreName=switch_t
  Data Store Write3 : DataStoreWrite  DataStoreName=FN
  Data Store Write4 : DataStoreWrite  DataStoreName=jRp
  Data Store Write5 : DataStoreWrite  DataStoreName=surf_num
  Data Store Write6 : DataStoreWrite  DataStoreName=reset_states
  Data Store Write7 : DataStoreWrite  DataStoreName=roll_reset_flag
  Demux : Demux  Outputs=[3;3]
  Integrator : Integrator  ExternalReset=level hold  InitialConditionSource=external  ShowStatePort=on
  Integrator1 : Integrator  ExternalReset=level hold  InitialConditionSource=external  ShowStatePort=on
  Integrator2 : Integrator  ExternalReset=level hold  InitialConditionSource=external  InitialCondition=[0;0;10]  ShowStatePort=on
  MATLAB Function : MATLAB Function  TreatAsAtomicUnit=on
  MATLAB Function1 : MATLAB Function  Priority=1  TreatAsAtomicUnit=on
  MATLAB Function11 : MATLAB Function  TreatAsAtomicUnit=on
  MATLAB Function2 : MATLAB Function  TreatAsAtomicUnit=on
  MATLAB Function3 : MATLAB Function  TreatAsAtomicUnit=on
  MATLAB Function4 : MATLAB Function  TreatAsAtomicUnit=on
  MATLAB Function5 : MATLAB Function  TreatAsAtomicUnit=on
  MATLAB Function6 : MATLAB Function  TreatAsAtomicUnit=on
  MATLAB Function7 : MATLAB Function  TreatAsAtomicUnit=on
  MATLAB Function8 : MATLAB Function  TreatAsAtomicUnit=on
  MATLAB Function9 : MATLAB Function  TreatAsAtomicUnit=on
  Mux : Mux  Inputs=[3;3;3;4]
  Mux1 : Mux  Inputs=[6;3;4]
  Scope : Scope
  Subsystem : Subsystem
  Subtract : Sum  Inputs=+-
  Switch{,1..3} (4 alike) : Switch  Criteria=u2 > Threshold
  Zero : Constant  Value=0  OutDataTypeStr=Inherit: Inherit via back propagation
  states : Outport
  inair_flag : Outport  Port=2  InitialOutput=1
  FW : Outport  Port=3
  wires:
  Data Store Read/1 -> MATLAB Function5/2(jAp)
  Mux/1 -> Switch3/1, MATLAB Function3/2(states), Switch1/1, MATLAB Function/1(states), Subsystem/2(states), MATLAB Function7/2(states), MATLAB Function4/1(states), MATLAB Function11/1(states)
  Data Store Read14/1 -> MATLAB Function5/9(rock_cents)
  MATLAB Function9/3(jR) -> Data Store Write4/1
  MATLAB Function5/3(q) -> Integrator1/3
  MATLAB Function5/5(reset_states) -> Data Store Write6/1
  Integrator/State -> Mux1/1
  MATLAB Function3/2(FN) -> Data Store Write3/1
  Subsystem/1(slip_flag) -> Scope/1, MATLAB Function7/11(slip_flag)
  Subsystem/5(FN) -> MATLAB Function7/12("FN ")
  Clock2/1 -> MATLAB Function5/1(t)
  MATLAB Function6/1(states0) -> MATLAB Function9/2(states)
  MATLAB Function5/6(surf_num) -> MATLAB Function2/4(surf_num), Data Store Write5/1
  Data Store Read18/1 -> MATLAB Function6/2(switch_t)
  Switch2/1 -> Data Store Write2/1
  Demux/1 -> Mux/1
  MATLAB Function8/1(O_v_TO) -> Mux/2
  Data Store Read13/1 -> MATLAB Function6/8("surf_num ")
  Data Store Read8/1 -> MATLAB Function6/6(rock_radi)
  MATLAB Function7/2(FN) -> MATLAB Function3/3("FN ")
  MATLAB Function7/1(angacc_linacc) -> Integrator/1
  MATLAB Function6/4(rock_coll_flag) -> MATLAB Function9/5(rock_coll_flag)
  Data Store Read19/1 -> MATLAB Function6/9(roll_reset_flag)
  Data Store Read3/1 -> MATLAB Function5/7(surf_num_memory)
  Data Store Read17/1 -> MATLAB Function6/4(states_from_memory)
  Subtract/1 -> Switch3/2
  Data Store Read11/1 -> MATLAB Function2/5(rock_cents)
  MATLAB Function4/1(q_dot) -> Integrator1/1
  Data Store Read16/1 -> MATLAB Function11/2(wv)
  MATLAB Function1/4(jA) -> Data Store Write/1
  MATLAB Function1/3(O_w_A) -> MATLAB Function8/3(O_w_A), MATLAB Function7/5(O_w_A), Subsystem/5(O_w_A)
  Data Store Read20/1 -> MATLAB Function6/10(reset_states)
  Data Store Read15/1 -> MATLAB Function5/10(rock_radi)
  Switch3/1 -> states/1
  Integrator1/State -> Mux1/3
  MATLAB Function6/5(surf_num) -> MATLAB Function5/8(surf_num_internal)
  Mux1/1 -> MATLAB Function6/3(states)
  MATLAB Function/1(slip_flag0) -> Subsystem/9(slip_flag0)
  Data Store Read10/1 -> MATLAB Function9/7(jRp)
  Data Store Read6/1 -> MATLAB Function5/11(switch_t)
  Integrator2/State -> Mux1/2
  Data Store Read21/1 -> MATLAB Function5/12("reset_states ")
  Data Store Read9/1 -> MATLAB Function6/5(rock_cents)
  MATLAB Function1/5(flag) -> Subsystem/1(flag)
  Integrator1/1 -> Mux/4  "q"
  Data Store Read5/1 -> MATLAB Function5/5("r_AO0 ")
  Subsystem/2(angacc_linacc) -> MATLAB Function7/1("angacc_linacc ")
  MATLAB Function9/1(states0) -> MATLAB Function5/4(states_internal)
  MATLAB Function5/1(OwT_OvAO0) -> Integrator/3
  MATLAB Function6/2(point_on_rock) -> MATLAB Function9/4(r_RO)
  Switch1/1 -> Data Store Write1/1
  Constant1/1 -> Switch3/3
  Subsystem/4(OalA_consts) -> MATLAB Function7/10(OalA_consts)
  MATLAB Function1/2(r_TO) -> Mux/3
  MATLAB Function3/1(inair_flag) -> Switch/1, Switch/2
  MATLAB Function6/3(rock_pardiffs) -> MATLAB Function9/6(rock_pardiffs)
  Integrator/1 -> Demux/1  "[OwT; OvAO]"
  Data Store Read1/1 -> MATLAB Function1/7(jAp)
  Zero/1 -> Switch/3
  Data Store Read7/1 -> MATLAB Function6/7(jAp)
  MATLAB Function9/2(roll_reset_flag) -> MATLAB Function5/6("roll_reset_flag ")
  Subsystem/3(OalA_coeffs) -> MATLAB Function7/9(OalA_coeffs)
  MATLAB Function5/4(roll_reset_flag) -> Integrator/2, MATLAB Function2/3(roll_reset_flag), Integrator1/2, Integrator2/2, Data Store Write7/1, MATLAB Function1/4(roll_reset_flag)
  "inputs "/1 -> Subsystem/3(inputs), MATLAB Function7/3(u), MATLAB Function9/3(u)
  Switch/1 -> Switch2/2, inair_flag/1, Switch1/2
  Clock/1 -> MATLAB Function9/1(t), MATLAB Function6/1(t), MATLAB Function1/1(t)
  Clock1/1 -> Subtract/1, Switch2/1
  MATLAB Function1/1(O_c_A) -> MATLAB Function3/1(O_c_A), MATLAB Function/2(O_c_A), MATLAB Function8/2(O_c_A), MATLAB Function7/4(O_c_A), Subsystem/4(O_c_A)
  Data Store Read2/1 -> Switch1/3, MATLAB Function5/3(states_from_memory)
  MATLAB Function11/1(FW) -> Subsystem/8(FW), MATLAB Function7/7(FW), FW/1
  Data Store Read4/1 -> Subtract/2, Switch2/3
  Demux/2 -> Subsystem/6(O_v_AO), MATLAB Function8/1(O_v_AO), MATLAB Function1/5(O_v_AO), MATLAB Function7/6(O_v_AO), Integrator2/1
  Integrator2/1 -> MATLAB Function2/1(r_AO), MATLAB Function1/2(r_AO)  "rAO"
  MATLAB Function2/1(par_diffs) -> Subsystem/7(par_diffs), MATLAB Function1/6(par_diffs), MATLAB Function7/8(par_diffs)
  MATLAB Function5/2(r_AO0) -> MATLAB Function2/2(r_AO0), MATLAB Function1/3(r_AO0), Integrator2/3

== system comprehensive_model_with_rocks_trial/bouncing_model/rockfield_gen ==
  states : Inport
  Clock : Clock
  Data Store Memory : DataStoreMemory  DataStoreName=set_sig  ReadBeforeWriteMsg=warning  WriteAfterWriteMsg=warning  WriteAfterReadMsg=warning  ShowAdditionalParam=off
  Data Store Memory1 : DataStoreMemory  DataStoreName=limit  ReadBeforeWriteMsg=warning  WriteAfterWriteMsg=warning  WriteAfterReadMsg=warning  ShowAdditionalParam=off
  Data Store Read : DataStoreRead  DataStoreName=rock_cents
  Data Store Read1 : DataStoreRead  DataStoreName=rock_radi
  Data Store Read2 : DataStoreRead  DataStoreName=set_sig
  Data Store Read3 : DataStoreRead  DataStoreName=limit
  Data Store Write : DataStoreWrite  DataStoreName=rock_cents
  Data Store Write1 : DataStoreWrite  DataStoreName=rock_radi
  Data Store Write2 : DataStoreWrite  DataStoreName=set_sig
  Data Store Write3 : DataStoreWrite  DataStoreName=limit
  MATLAB Function1 : MATLAB Function  TreatAsAtomicUnit=on
  Random Number : RandomNumber  Mean=0.25*ones(50,1)  Variance=0.15*ones(50,1)  Seed=randi(100,50,1)  SampleTime=0.01  VectorParams1D=off
  Uniform Random Number : UniformRandomNumber  Minimum=0*ones(3,50)  Maximum=1*ones(3,50)  Seed=randi(100,3,50)  SampleTime=0.01  VectorParams1D=off
  wires:
  Uniform Random Number/1 -> MATLAB Function1/3(rockcent_rand)
  Random Number/1 -> MATLAB Function1/4(rockrad_rand)
  Data Store Read/1 -> MATLAB Function1/5("rock_cents ")
  MATLAB Function1/1(rock_cents) -> Data Store Write/1
  Data Store Read1/1 -> MATLAB Function1/6("rock_radi ")
  MATLAB Function1/2(rock_radi) -> Data Store Write1/1
  Clock/1 -> MATLAB Function1/1(t)
  states/1 -> MATLAB Function1/2(states)
  Data Store Read2/1 -> MATLAB Function1/7("set_sig ")
  Data Store Read3/1 -> MATLAB Function1/8("limit ")
  MATLAB Function1/3(set_sig) -> Data Store Write2/1
  MATLAB Function1/4(limit) -> Data Store Write3/1

== system comprehensive_model_with_rocks_trial/bouncing_model/rockfield_gen1 ==
  states : Inport
  Clock : Clock
  Data Store Memory : DataStoreMemory  DataStoreName=set_sig  ReadBeforeWriteMsg=warning  WriteAfterWriteMsg=warning  WriteAfterReadMsg=warning  ShowAdditionalParam=off
  Data Store Memory1 : DataStoreMemory  DataStoreName=limit  ReadBeforeWriteMsg=warning  WriteAfterWriteMsg=warning  WriteAfterReadMsg=warning  ShowAdditionalParam=off
  Data Store Memory2 : DataStoreMemory  DataStoreName=all_rock_cents  ReadBeforeWriteMsg=warning  WriteAfterWriteMsg=warning  WriteAfterReadMsg=warning  InitialValue=rc2  ShowAdditionalParam=off
  Data Store Memory3 : DataStoreMemory  DataStoreName=all_rock_rads  ReadBeforeWriteMsg=warning  WriteAfterWriteMsg=warning  WriteAfterReadMsg=warning  InitialValue=rr2  ShowAdditionalParam=off
  Data Store Read : DataStoreRead  DataStoreName=rock_cents
  Data Store Read1 : DataStoreRead  DataStoreName=rock_radi
  Data Store Read2 : DataStoreRead  DataStoreName=set_sig
  Data Store Read3 : DataStoreRead  DataStoreName=limit
  Data Store Read4 : DataStoreRead  DataStoreName=all_rock_cents
  Data Store Read5 : DataStoreRead  DataStoreName=all_rock_rads
  Data Store Write : DataStoreWrite  DataStoreName=rock_cents
  Data Store Write1 : DataStoreWrite  DataStoreName=rock_radi
  Data Store Write2 : DataStoreWrite  DataStoreName=set_sig
  Data Store Write3 : DataStoreWrite  DataStoreName=limit
  MATLAB Function1 : MATLAB Function  TreatAsAtomicUnit=on
  wires:
  Data Store Read/1 -> MATLAB Function1/3("rock_cents ")
  MATLAB Function1/1(rock_cents) -> Data Store Write/1
  Data Store Read1/1 -> MATLAB Function1/4("rock_radi ")
  MATLAB Function1/2(rock_radi) -> Data Store Write1/1
  Clock/1 -> MATLAB Function1/1(t)
  states/1 -> MATLAB Function1/2(states)
  Data Store Read2/1 -> MATLAB Function1/5("set_sig ")
  Data Store Read3/1 -> MATLAB Function1/6("limit ")
  MATLAB Function1/3(set_sig) -> Data Store Write2/1
  MATLAB Function1/4(limit) -> Data Store Write3/1
  Data Store Read4/1 -> MATLAB Function1/8(all_rock_cents)
  Data Store Read5/1 -> MATLAB Function1/7(all_rock_rads)

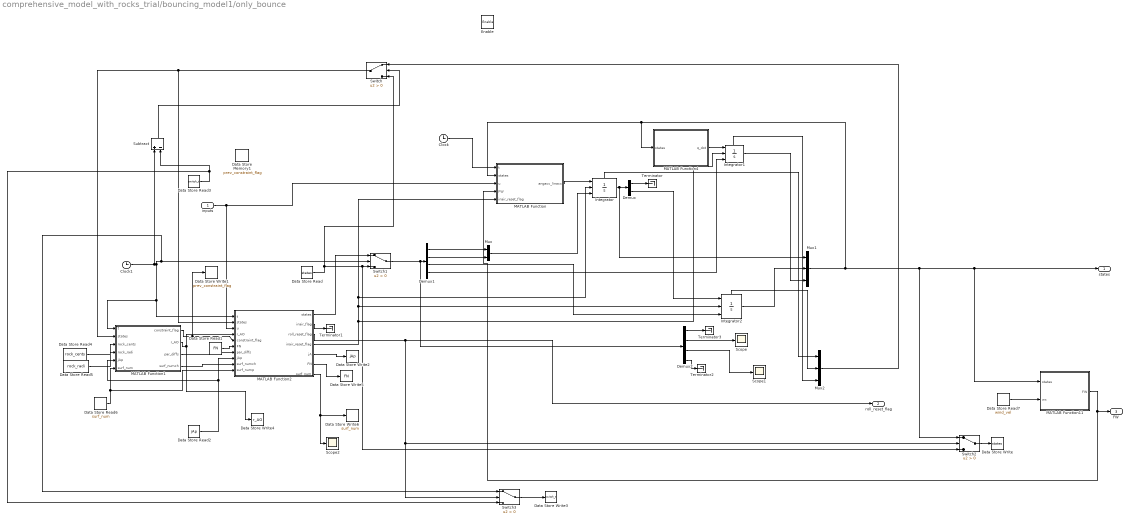
== system comprehensive_model_with_rocks_trial/bouncing_model1/only_bounce ==
  inputs : Inport
  Enable : EnablePort  StatesWhenEnabling=reset
  Clock : Clock
  Clock1 : Clock
  Data Store Memory1 : DataStoreMemory  DataStoreName=prev_constraint_flag  ReadBeforeWriteMsg=warning  WriteAfterWriteMsg=warning  WriteAfterReadMsg=warning  ShowAdditionalParam=off
  Data Store Read : DataStoreRead  DataStoreName=states
  Data Store Read1 : DataStoreRead  DataStoreName=FN
  Data Store Read2 : DataStoreRead  DataStoreName=jAp
  Data Store Read3 : DataStoreRead  DataStoreName=switch_t
  Data Store Read4 : DataStoreRead  DataStoreName=rock_cents
  Data Store Read5 : DataStoreRead  DataStoreName=rock_radi
  Data Store Read6 : DataStoreRead  DataStoreName=surf_num
  Data Store Read7 : DataStoreRead  DataStoreName=wind_vel
  Data Store Write : DataStoreWrite  DataStoreName=states
  Data Store Write1 : DataStoreWrite  DataStoreName=prev_constraint_flag
  Data Store Write2 : DataStoreWrite  DataStoreName=jAp
  Data Store Write3 : DataStoreWrite  DataStoreName=switch_t
  Data Store Write4 : DataStoreWrite  DataStoreName=r_AO
  Data Store Write5 : DataStoreWrite  DataStoreName=FN
  Data Store Write6 : DataStoreWrite  DataStoreName=surf_num
  Demux : Demux  Outputs=[3;3]
  Demux1 : Demux  Outputs=[3;3;3;4]
  Demux2 : Demux  Outputs=[3;3;3;4]
  Integrator : Integrator  ExternalReset=level hold  InitialConditionSource=external  ShowStatePort=on
  Integrator1 : Integrator  ExternalReset=level hold  InitialConditionSource=external  ShowStatePort=on
  Integrator2 : Integrator  ExternalReset=level hold  InitialConditionSource=external  ShowStatePort=on
  MATLAB Function : MATLAB Function  TreatAsAtomicUnit=on
  MATLAB Function1 : MATLAB Function  TreatAsAtomicUnit=on
  MATLAB Function11 : MATLAB Function  TreatAsAtomicUnit=on
  MATLAB Function2 : MATLAB Function  TreatAsAtomicUnit=on
  MATLAB Function4 : MATLAB Function  TreatAsAtomicUnit=on
  Mux : Mux  Inputs=2
  Mux1 : Mux  Inputs=[6;3;4]
  Mux2 : Mux  Inputs=[6;3;4]
  Scope : Scope
  Scope1 : Scope
  Scope2 : Scope
  Subtract : Sum  Inputs=+-
  Switch{,1..3} (4 alike) : Switch  Criteria=u2 > Threshold
  Terminator{,1..3} (4 alike) : Terminator
  states : Outport  SourceOfInitialOutputValue=Input signal  InitialOutput=zeros(13,1)
  roll_reset_flag : Outport  Port=2  InitialOutput=0
  FW : Outport  Port=3
  wires:
  Integrator2/State -> Mux2/2
  MATLAB Function2/5(jA) -> Data Store Write2/1
  MATLAB Function2/2(inair_flag) -> Terminator1/1
  MATLAB Function1/2(r_AO) -> Data Store Write4/1, MATLAB Function2/4(r_AO)
  Clock1/1 -> Subtract/1, Switch1/2, Switch3/1, MATLAB Function1/1(t), MATLAB Function2/1(t)
  MATLAB Function1/1(constraint_flag) -> MATLAB Function2/5(constraint_flag), Data Store Write1/1
  Integrator/State -> Mux2/1
  MATLAB Function4/1(q_dot) -> Integrator1/1
  Mux1/1 -> MATLAB Function4/1(states), MATLAB Function/2(states), Switch2/1, MATLAB Function11/1(states), states/1
  Integrator1/1 -> Mux1/3
  Clock/1 -> MATLAB Function/1(t)
  Demux2/1 -> Terminator3/1
  Integrator/1 -> Mux1/1, Demux/1
  Demux2/4 -> Terminator2/1
  Demux1/2 -> Mux/2
  inputs/1 -> MATLAB Function/3(u), MATLAB Function2/3(u)
  MATLAB Function1/3(par_diffs) -> MATLAB Function2/7(par_diffs)
  Demux1/4 -> Integrator1/3
  Demux/1 -> Terminator/1
  Demux2/3 -> Scope1/1
  Demux/2 -> Integrator2/1
  Demux2/2 -> Scope/1
  Integrator1/State -> Mux2/3
  Mux/1 -> Integrator/3
  Demux1/1 -> Mux/1
  MATLAB Function2/4(inair_reset_flag) -> Integrator/2, MATLAB Function/5(inair_reset_flag), Integrator2/2, Integrator1/2
  MATLAB Function11/1(FW) -> FW/1, MATLAB Function/4(FW)
  MATLAB Function/1(angacc_linacc) -> Integrator/1
  Demux1/3 -> Integrator2/3
  Integrator2/1 -> Mux1/2
  Data Store Read2/1 -> MATLAB Function1/5(jAp), MATLAB Function2/8(jAp)
  Mux2/1 -> Switch/1
  Switch/1 -> MATLAB Function2/2("states "), MATLAB Function1/2(states)
  Switch1/1 -> Demux2/1, Demux1/1
  MATLAB Function2/1(states) -> Switch1/1
  Data Store Read/1 -> Switch/3, Switch2/3, Switch1/3
  Switch2/1 -> Data Store Write/1
  Data Store Read3/1 -> Switch3/3, Subtract/2
  Subtract/1 -> Switch/2
  Switch3/1 -> Data Store Write3/1
  MATLAB Function2/3(roll_reset_flag) -> roll_reset_flag/1, Switch2/2, Switch3/2
  Data Store Read1/1 -> MATLAB Function2/6("FN ")
  MATLAB Function2/6(FN) -> Data Store Write5/1
  Data Store Read4/1 -> MATLAB Function1/3(rock_cents)
  Data Store Read5/1 -> MATLAB Function1/4(rock_radi)
  MATLAB Function1/4(surf_numch) -> MATLAB Function2/9(surf_numch)
  MATLAB Function2/7(surf_num) -> Scope2/1, Data Store Write6/1
  Data Store Read6/1 -> MATLAB Function2/10(surf_nump), MATLAB Function1/6(surf_num)
  Data Store Read7/1 -> MATLAB Function11/2(wx)
